simulink model "GFLIB_AtanYXShifted_BAM_FLT"  (Simulink 8.3)
settings: Solver=ode45  StartTime=0.0  StopTime=10.0  RelTol=1e-3
undefined symbols (not defined in the file): Kx, Ky, ThetaAdj
settings Model: Creator=RE004C  LastModifiedBy=B17364
settings OptimizationCC: ExpressionDepthLimit=2147483647
settings DebuggingCC: FcnCallInpInsideContextMsg=UseLocalSettings  StrictBusMsg=Warning
settings HardwareCC: ProdLargestAtomicInteger=Long  ProdLargestAtomicFloat=Double  ProdIntDivRoundTo=Zero  ProdEndianess=BigEndian  ProdHWDeviceType=Freescale->32-bit PowerPC

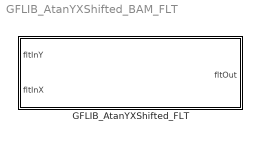
== system GFLIB_AtanYXShifted_BAM_FLT ==
  GFLIB_AtanYXShifted_FLT : Subsystem  mask(GFLIB_AtanYXShifted_FLT){Ky=Ky, Kx=Kx, ThetaAdj=ThetaAdj}
      mask help: Bit accurate model of GFLIB_AtanYXShifted function.
      mask init:
      | pos = get_param(gcb, 'Position');width = pos(3) - pos(1); height = pos(4) - pos(2);tX=width/2;tY=height*0.9;
      mask Display: color('black');port_label('input',1,'fltInY');port_label('input',2,'fltInX');port_label('output',1,'fltOut');color('black');disp('GFLIB_AtanYXShifted_FLT');color('blue');text(tX,tY, 'BAM', 'horizontalAlignment', 'center');

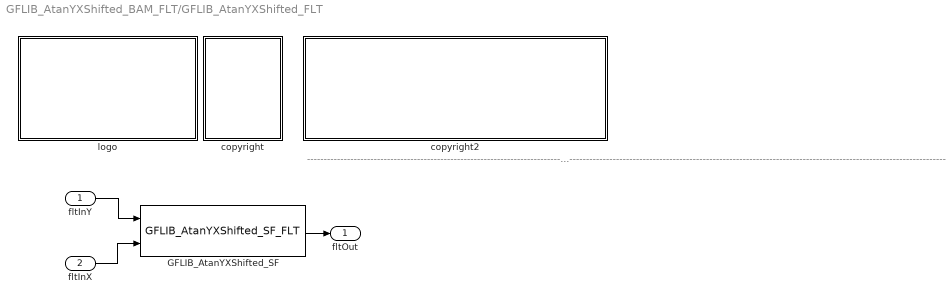
== system GFLIB_AtanYXShifted_BAM_FLT/GFLIB_AtanYXShifted_FLT ==
  note: ---------------------------------------------------------------------------------------------------------------------------------------------------------------------------------------------------
  fltInY : Inport
  fltInX : Inport  Port=2
  GFLIB_AtanYXShifted_SF : S-Function  FunctionName=GFLIB_AtanYXShifted_SF_FLT  Parameters=Ky,Kx,ThetaAdj  EnableBusSupport=off
  copyright : Subsystem
      mask Display:
      | text(10,90,'FILE:');text(10,75,'DESRIPTION:')
      | text(10,60,'COPYRIGHT:')
      | text(10,45,'VERSION:')
      | text(10,30,'DATE:')
  copyright2 : Subsystem
      mask Display:
      | text(10,90,'GFLIB_AtanYXShifted_BAM_FLT.mdl');text(10,75,'Shifted YX Arctangent of argument.');text(10,60,'Freescale')
      | text(10,45,'0.1');text(10,30,'06-Sep-2011');
  logo : Subsystem
      mask Display: image(imread('logo.jpg'))
  fltOut : Outport
  wires:
  fltInY/1 -> GFLIB_AtanYXShifted_SF/1
  fltInX/1 -> GFLIB_AtanYXShifted_SF/2
  GFLIB_AtanYXShifted_SF/1 -> fltOut/1

== system GFLIB_AtanYXShifted_BAM_FLT/GFLIB_AtanYXShifted_FLT/copyright ==

== system GFLIB_AtanYXShifted_BAM_FLT/GFLIB_AtanYXShifted_FLT/copyright2 ==

== system GFLIB_AtanYXShifted_BAM_FLT/GFLIB_AtanYXShifted_FLT/logo ==
